simulink model "untitled1"  (R2018b)
settings: Solver=VariableStepAuto  StartTime=0.0  StopTime=3  RelTol=1e-3
libraries: commfilt2 x2, dsparch4 x1, commsink2 x1, commutil2 x1, commrandsrc3 x1
settings Model: Creator=nhat  LastModifiedBy=nhat

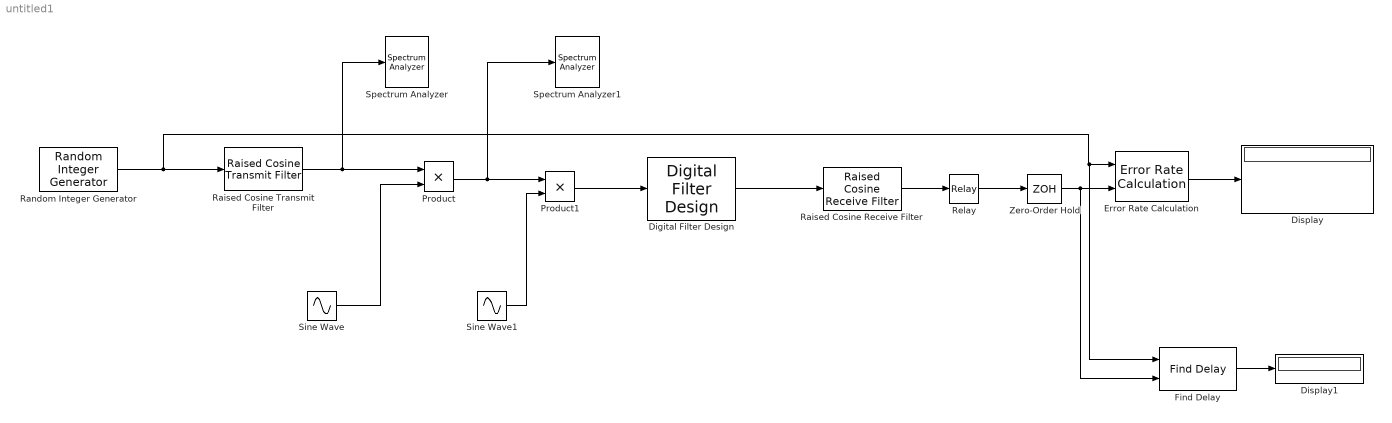
== system untitled1 ==
  Digital Filter Design : dsparch4/Digital Filter Design  mwdsp_browser_bugfix_var=off
  Display : Display
  Display1 : Display
  Error Rate Calculation : commsink2/Error Rate Calculation  N=6  st_delay=0  cp_mode=Entire frame  subframe=[]  PMode=Port  WsName=ErrorVec  RsMode2=off  stop=off  numErr=100  maxBits=1e6
  Find Delay : commutil2/Find Delay  corrLength=200  chgSigOP=off  stopUpdate=off  numConstDelay=3
      settings: SourceProductName=Communications System Toolbox  SourceProductBaseCode=CM
  Product : Product
  Product1 : Product
  Raised Cosine Receive Filter : commfilt2/Raised Cosine Receive Filter  filtType=Square root  R=1  filtSpan=10  N=10  downFactor=10  downOffset=3  filterGain=1  RateOptions=Allow multirate processing  framing=Mute  checkCoeff=off  variableName=rcRxFilt  currentFiltSpan=10  D=5  inputOffset=0  sampMode=Mute  saveAsFlag=0  rateMode=Downsampling  checkGain=Normalized  launchFVT=on  roundingMode=Floor  overflowMode=off  coeffDataTypeStr=Inherit: Same word length as input  coeffMin=[]  coeffMax=[]  coeffLastDataTypeStr=Inherit: Same word length as input  accumDataTypeStr=Inherit: Same as product output  accumLastDataTypeStr=Inherit: Same as product output  outputDataTypeStr=Inherit: Same as accumulator  outputMin=[]  outputMax=[]  outputLastDataTypeStr=Inherit: Same as accumulator
  Raised Cosine Transmit Filter : commfilt2/Raised Cosine Transmit Filter  filtType=Square root  R=1  filtSpan=10  N=10  filterGain=1  RateOptions=Allow multirate processing  framing=Mute  checkCoeff=off  variableName=rcTxFilt  checkGain=Normalized  sampMode=Mute  saveAsFlag=0  currentFiltSpan=10  D=5  launchFVT=on  roundingMode=Floor  overflowMode=off  coeffDataTypeStr=Inherit: Same word length as input  coeffMin=[]  coeffMax=[]  coeffLastDataTypeStr=Inherit: Same word length as input  outputDataTypeStr=Inherit: Same as accumulator  outputMin=[]  outputMax=[]  outputLastDataTypeStr=Inherit: Same as accumulator
  Random Integer Generator : commrandsrc3/Random Integer Generator  SetSize=2  SeedSource=Auto  Seed=0  SampleTime=1/1000  SamplesPerFrame=1  OutputDataType=double  SimulateUsing=Interpreted execution
  Relay : Relay  OnSwitchValue=0.3  OffSwitchValue=0.2
  Sine Wave : Sin  Frequency=10000*2*pi  SampleTime=1/100000
  Sine Wave1 : Sin  Frequency=10000*2*pi  SampleTime=1/100000
  Spectrum Analyzer : SpectrumAnalyzer
  Spectrum Analyzer1 : SpectrumAnalyzer
  Zero-Order Hold : ZeroOrderHold  SampleTime=1/1000
  wires:
  Random Integer Generator/1 -> Raised Cosine Transmit Filter/1, Find Delay/1, Error Rate Calculation/1
  Raised Cosine Transmit Filter/1 -> Spectrum Analyzer/1, Product/1
  Product/1 -> Spectrum Analyzer1/1, Product1/1
  Product1/1 -> Digital Filter Design/1
  Digital Filter Design/1 -> Raised Cosine Receive Filter/1
  Raised Cosine Receive Filter/1 -> Relay/1
  Relay/1 -> Zero-Order Hold/1
  Zero-Order Hold/1 -> Find Delay/2, Error Rate Calculation/2
  Error Rate Calculation/1 -> Display/1
  Sine Wave/1 -> Product/2
  Sine Wave1/1 -> Product1/2
  Find Delay/1 -> Display1/1
